simulink model "AdaptiveModel"  (R2016b)
settings: Solver=VariableStepAuto  StartTime=0.0  StopTime=10.0  RelTol=1e-3
values from neighbouring files (symbols this model uses):
  d = 1    [main.m]
  nA = length(A1)-1    [LPV_Torsional.m]    (also in main.m = length(G1.f)-1)
  nB = length(B1)-1    [LPV_Torsional.m]    (also in main.m = length(G1.b)-1-d)
settings Model: Creator=akarimi  LastModifiedBy=akarimi

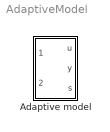
== system AdaptiveModel ==
  Adaptive model : Subsystem

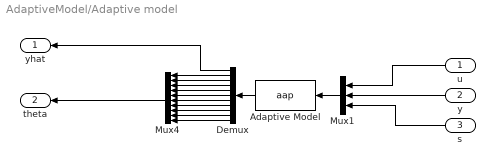
== system AdaptiveModel/Adaptive model ==
  u : Inport
  y : Inport  Port=2
  s : Inport  Port=3
  "Adaptive Model " : S-Function  FunctionName=aap  Parameters=nA,nB,d  SFunctionDeploymentMode=off  EnableBusSupport=off
  Demux : Demux  Outputs=11
  Mux1 : Mux  Inputs=3
  Mux4 : Mux  Inputs=10
  yhat : Outport
  theta : Outport  Port=2
  wires:
  Mux1/1 -> "Adaptive Model "/1
  "Adaptive Model "/1 -> Demux/1
  Demux/1 -> yhat/1
  Mux4/1 -> theta/1
  Demux/2 -> Mux4/1
  Demux/3 -> Mux4/2
  Demux/4 -> Mux4/3
  Demux/5 -> Mux4/4
  Demux/6 -> Mux4/5
  Demux/7 -> Mux4/6
  Demux/8 -> Mux4/7
  Demux/9 -> Mux4/8
  Demux/10 -> Mux4/9
  Demux/11 -> Mux4/10
  u/1 -> Mux1/1
  y/1 -> Mux1/2
  s/1 -> Mux1/3
